simulink model "PreventOversaturationTest"  (R2025b)
settings: Solver=VariableStepAuto  StartTime=0.0  StopTime=10.0  RelTol=1e-3
libraries: Bibliothek_FHDO_V1 x7, simulink x1
settings Model: Creator=goessling  LastModifiedBy=goessling

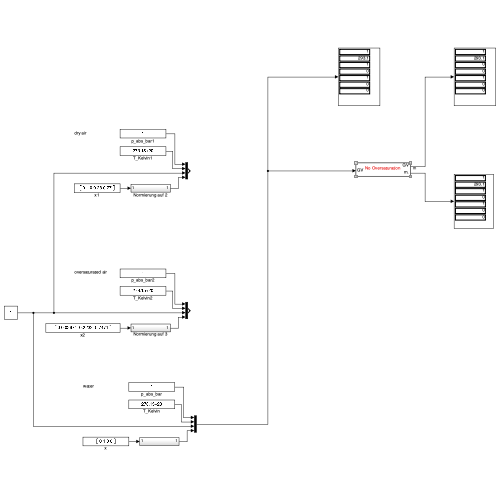
[thumbnail: Simulink's stored preview of the top-level diagram]
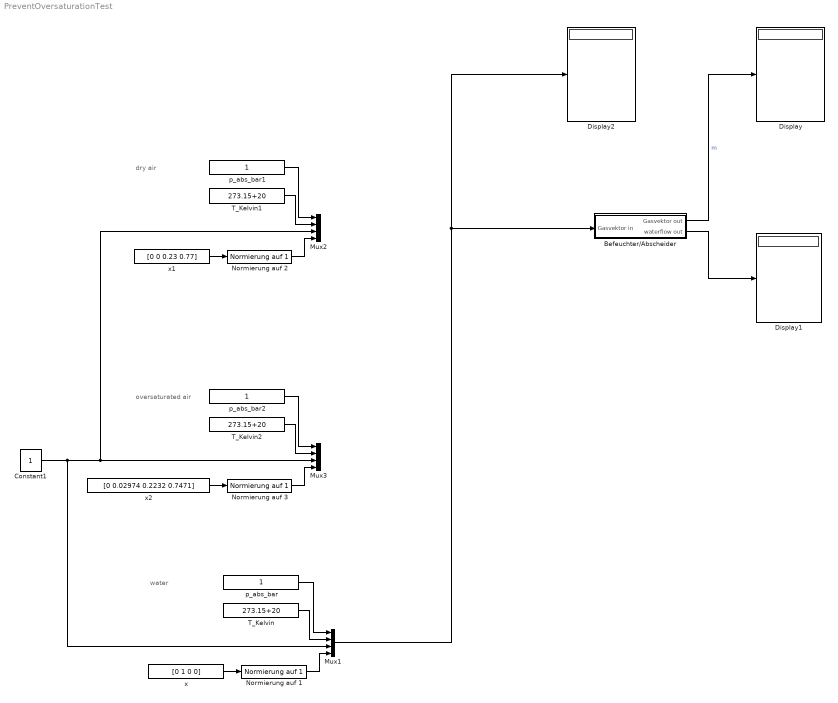
== system PreventOversaturationTest ==
  note: dry air
  note: oversaturated air
  note: water
  Befeuchter/Abscheider : Subsystem
      mask Display:
      | color('red')
      | disp('No Oversaturation');
      | 
      | color('black')
      | port_label('output', 1, 'GV')
      | port_label('output', 2, 'm.')
      | port_label('input', 1, 'GV')
  Constant1 : Constant
  Display : Display
  Display1 : Display
  Display2 : Display
  Mux1 : Mux
  Mux2 : Mux
  Mux3 : Mux
  Normierung auf 1 : Bibliothek_FHDO_V1/Wasser/Normierung auf 1  SystemSampleTime=-1  VariantActivationTime=update diagram  EmptyChoice=off  PassThrough=off  PassThroughVariantControl=(default)  EmptyChoiceVariantControl=(default)  AllowFlexibleInterface=on  Latency=0  AutoFrameSizeCalculation=off
  Normierung auf 2 : Bibliothek_FHDO_V1/Wasser/Normierung auf 1  SystemSampleTime=-1  VariantActivationTime=update diagram  EmptyChoice=off  PassThrough=off  PassThroughVariantControl=(default)  EmptyChoiceVariantControl=(default)  AllowFlexibleInterface=on  Latency=0  AutoFrameSizeCalculation=off
  Normierung auf 3 : Bibliothek_FHDO_V1/Wasser/Normierung auf 1  SystemSampleTime=-1  VariantActivationTime=update diagram  EmptyChoice=off  PassThrough=off  PassThroughVariantControl=(default)  EmptyChoiceVariantControl=(default)  AllowFlexibleInterface=on  Latency=0  AutoFrameSizeCalculation=off
  T_Kelvin : Constant  Value=273.15+20
  T_Kelvin1 : Constant  Value=273.15+20
  T_Kelvin2 : Constant  Value=273.15+20
  p_abs_bar : Constant
  p_abs_bar1 : Constant
  p_abs_bar2 : Constant
  x : Constant  Value=[0 1 0 0]
  x1 : Constant  Value=[0 0 0.23 0.77]
  x2 : Constant  Value=[0 0.02974 0.2232 0.7471]
  wires:
  Normierung auf 3/1 -> Mux3/4
  p_abs_bar2/1 -> Mux3/1
  T_Kelvin1/1 -> Mux2/2
  p_abs_bar1/1 -> Mux2/1
  Normierung auf 2/1 -> Mux2/4
  x1/1 -> Normierung auf 2/1
  T_Kelvin2/1 -> Mux3/2
  x2/1 -> Normierung auf 3/1
  Befeuchter/Abscheider/1(Gasvektor out) -> Display/1  "m"
  Befeuchter/Abscheider/2(waterflow out) -> Display1/1
  Normierung auf 1/1 -> Mux1/4
  T_Kelvin/1 -> Mux1/2
  p_abs_bar/1 -> Mux1/1
  Constant1/1 -> Mux1/3, Mux2/3, Mux3/3
  x/1 -> Normierung auf 1/1
  Mux1/1 -> Befeuchter/Abscheider/1(Gasvektor in), Display2/1

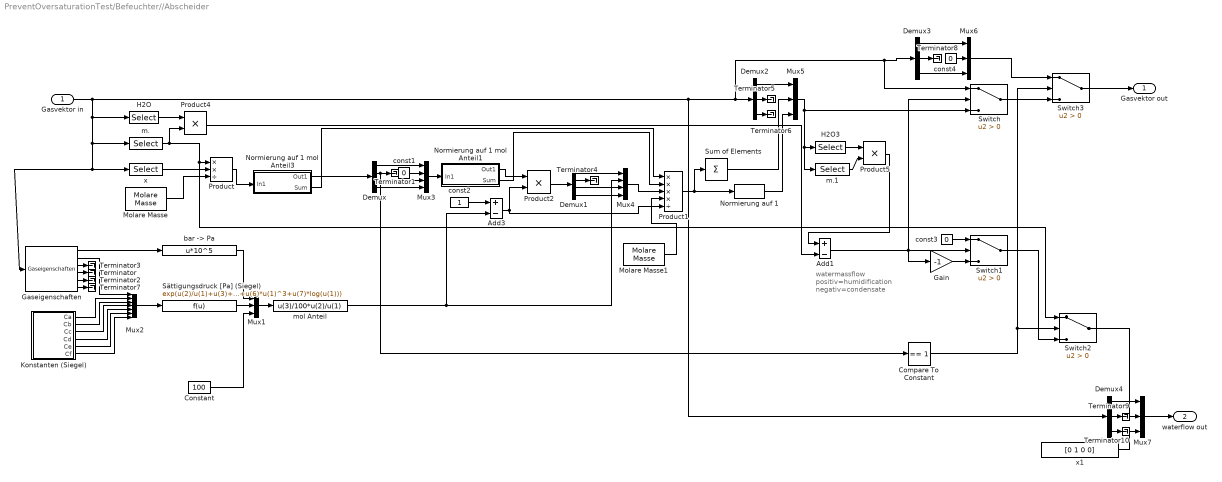
== system PreventOversaturationTest/Befeuchter//Abscheider ==
  note: watermassflow
      | positiv=humidification
      | negativ=condensate
  Gasvektor in : Inport
  Add1 : Sum  Inputs=+-
  Add3 : Sum  Inputs=+-
  Compare To Constant : simulink/Logic and Bit Operations/Compare To Constant  relop===  const=1  OutDataTypeStr=boolean
  Constant : Constant  Value=100
  Demux : Demux
  Demux1 : Demux
  Demux2 : Demux  Outputs=[2 1 4]
  Demux3 : Demux  Outputs=[2 1 4]
  Demux4 : Demux  Outputs=[2 1 4]
  Gain : Gain  Gain=-1
  Gaseigenschaften : Bibliothek_FHDO_V1/Gaseigenschaften  SystemSampleTime=-1  VariantActivationTime=update diagram  EmptyChoice=off  PassThrough=off  PassThroughVariantControl=(default)  EmptyChoiceVariantControl=(default)  AllowFlexibleInterface=on  Latency=0  AutoFrameSizeCalculation=off
  H2O : Selector  InputPortWidth=7  IndexOptions=Index vector (dialog)  Indices=5  OutputSizes=1
  H2O3 : Selector  InputPortWidth=7  IndexOptions=Index vector (dialog)  Indices=5  OutputSizes=1
  Konstanten (Siegel) : Subsystem
  Molare Masse : Bibliothek_FHDO_V1/Molare Masse  SystemSampleTime=-1  VariantActivationTime=update diagram  EmptyChoice=off  PassThrough=off  PassThroughVariantControl=(default)  EmptyChoiceVariantControl=(default)  AllowFlexibleInterface=on  Latency=0  AutoFrameSizeCalculation=off
  Molare Masse1 : Bibliothek_FHDO_V1/Molare Masse  SystemSampleTime=-1  VariantActivationTime=update diagram  EmptyChoice=off  PassThrough=off  PassThroughVariantControl=(default)  EmptyChoiceVariantControl=(default)  AllowFlexibleInterface=on  Latency=0  AutoFrameSizeCalculation=off
  Mux{1,5..7} (4 alike) : Mux  Inputs=3
  Mux2 : Mux  Inputs=7
  Mux3 : Mux
  Mux4 : Mux
  Normierung auf 1 : Bibliothek_FHDO_V1/Sauerstoff/Normierung auf 1  SystemSampleTime=-1  VariantActivationTime=update diagram  EmptyChoice=off  PassThrough=off  PassThroughVariantControl=(default)  EmptyChoiceVariantControl=(default)  AllowFlexibleInterface=on  Latency=0  AutoFrameSizeCalculation=off
  Normierung auf 1 mol Anteil1 : Subsystem
  Normierung auf 1 mol Anteil3 : Subsystem
  Product : Product  Inputs=**/  RndMeth=Zero
  Product1 : Product  Inputs=****/  RndMeth=Zero
  Product2 : Product  RndMeth=Zero
  Product4 : Product  RndMeth=Zero
  Product5 : Product  RndMeth=Zero
  Sum of Elements : Sum  Inputs=+
  Switch{,1..3} (4 alike) : Switch  Criteria=u2 > Threshold  SaturateOnIntegerOverflow=off  InputSameDT=off
  Sättigungsdruck [Pa] (Siegel) : Fcn  Expr=exp(u(2)/u(1)+u(3)+u(4)*u(1)+u(5)*u(1)^2+u(6)*u(1)^3+u(7)*log(u(1)))
  Terminator{,1..10} (11 alike) : Terminator
  "bar -> Pa" : Fcn  Expr=u*10^5
  const1 : Constant  Value=0
  const2 : Constant
  const3 : Constant  Value=0
  const4 : Constant  Value=0
  m. : Selector  InputPortWidth=7  IndexOptions=Index vector (dialog)  Indices=3  OutputSizes=1
  m.1 : Selector  InputPortWidth=7  IndexOptions=Index vector (dialog)  Indices=3  OutputSizes=1
  mol Anteil : Fcn  Expr=u(3)/100*u(2)/u(1)
  x : Selector  InputPortWidth=7  IndexOptions=Index vector (dialog)  Indices=[4 5 6 7]  OutputSizes=1
  x1 : Constant  Value=[0 1 0 0]
  Gasvektor out : Outport
  waterflow out : Outport  Port=2
  wires:
  Demux1/4 -> Mux4/4
  Demux1/3 -> Mux4/3
  Demux1/1 -> Mux4/1
  Demux1/2 -> Terminator4/1
  Demux/4 -> Mux3/4
  Demux/3 -> Mux3/3
  Demux/1 -> Mux3/1
  const1/1 -> Mux3/2
  Demux/2 -> Compare To Constant/1, Terminator1/1
  Product4/1 -> Add1/2
  Product5/1 -> Add1/1
  H2O3/1 -> Product5/1
  m.1/1 -> Product5/2
  H2O/1 -> Product4/1
  Normierung auf 1 mol Anteil1/2(Sum) -> Product1/2
  Normierung auf 1 mol Anteil3/2(Sum) -> Product1/1
  Normierung auf 1 mol Anteil3/1(Out1) -> Demux/1
  Normierung auf 1/1 -> Mux5/3
  Mux5/1 -> Switch/3, m.1/1, H2O3/1
  Demux2/3 -> Terminator6/1
  Demux2/2 -> Terminator5/1
  Product1/1 -> Normierung auf 1/1, Sum of Elements/1
  Sum of Elements/1 -> Mux5/2
  Demux2/1 -> Mux5/1
  m./1 -> Switch2/1, Product/1, Product4/2
  Molare Masse1/1 -> Product1/4
  Mux4/1 -> Product1/3
  Product2/1 -> Demux1/1
  Add3/1 -> Product1/5, Product2/2
  Normierung auf 1 mol Anteil1/1(Out1) -> Product2/1
  mol Anteil/1 -> Mux4/2, Add3/2
  const2/1 -> Add3/1
  Mux3/1 -> Normierung auf 1 mol Anteil1/1(In1)
  Product/1 -> Normierung auf 1 mol Anteil3/1(In1)
  Molare Masse/1 -> Product/3
  x/1 -> Product/2
  "bar -> Pa"/1 -> Mux1/1
  Constant/1 -> Mux1/3
  Mux1/1 -> mol Anteil/1
  Sättigungsdruck [Pa] (Siegel)/1 -> Mux1/2
  Mux2/1 -> Sättigungsdruck [Pa] (Siegel)/1
  Gaseigenschaften/5 -> Terminator2/1
  Gaseigenschaften/4 -> Terminator/1
  Gaseigenschaften/3 -> Terminator3/1
  Gaseigenschaften/1 -> "bar -> Pa"/1
  Konstanten (Siegel)/6(Cf) -> Mux2/7
  Konstanten (Siegel)/5(Ce) -> Mux2/6
  Konstanten (Siegel)/4(Cd) -> Mux2/5
  Konstanten (Siegel)/3(Cc) -> Mux2/4
  Konstanten (Siegel)/2(Cb) -> Mux2/3
  Konstanten (Siegel)/1(Ca) -> Mux2/2
  Gaseigenschaften/2 -> Mux2/1
  Gasvektor in/1 -> Demux3/1, Switch/1, Demux2/1, Demux4/1, H2O/1, Gaseigenschaften/1, x/1, m./1
  Gaseigenschaften/6 -> Terminator7/1
  Add1/1 -> Gain/1, Switch1/2, Switch/2
  Switch/1 -> Switch3/3
  const3/1 -> Switch1/1
  Compare To Constant/1 -> Switch3/2, Switch2/2
  Switch2/1 -> Mux7/2
  Switch1/1 -> Switch2/3
  Demux3/1 -> Mux6/1
  Demux3/3 -> Mux6/3
  const4/1 -> Mux6/2
  Demux3/2 -> Terminator8/1
  Mux6/1 -> Switch3/1
  Switch3/1 -> Gasvektor out/1
  Demux4/1 -> Mux7/1
  Demux4/2 -> Terminator9/1
  Demux4/3 -> Terminator10/1
  x1/1 -> Mux7/3
  Mux7/1 -> waterflow out/1
  Gain/1 -> Switch1/3

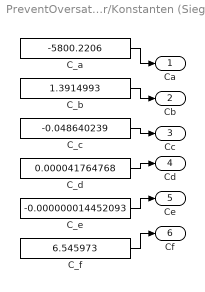
== system PreventOversaturationTest/Befeuchter//Abscheider/Konstanten (Siegel) ==
  C_a : Constant  Value=-5800.2206
  C_b : Constant  Value=1.3914993
  C_c : Constant  Value=-0.048640239
  C_d : Constant  Value=0.000041764768
  C_e : Constant  Value=-0.000000014452093
  C_f : Constant  Value=6.545973
  Ca : Outport
  Cb : Outport  Port=2
  Cc : Outport  Port=3
  Cd : Outport  Port=4
  Ce : Outport  Port=5
  Cf : Outport  Port=6
  wires:
  C_f/1 -> Cf/1
  C_e/1 -> Ce/1
  C_d/1 -> Cd/1
  C_c/1 -> Cc/1
  C_b/1 -> Cb/1
  C_a/1 -> Ca/1

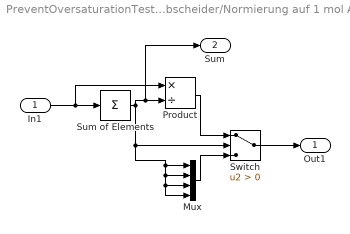
== system PreventOversaturationTest/Befeuchter//Abscheider/Normierung auf 1 mol Anteil1 ==
  In1 : Inport
  Mux : Mux
  Product : Product  Inputs=*/  RndMeth=Zero
  Sum of Elements : Sum  Inputs=+
  Switch : Switch  Criteria=u2 > Threshold  SaturateOnIntegerOverflow=off  InputSameDT=off
  Out1 : Outport
  Sum : Outport  Port=2
  wires:
  In1/1 -> Sum of Elements/1, Product/1
  Sum of Elements/1 -> Switch/2, Mux/4, Mux/3, Mux/2, Mux/1, Product/2, Sum/1
  Product/1 -> Switch/1
  Switch/1 -> Out1/1
  Mux/1 -> Switch/3

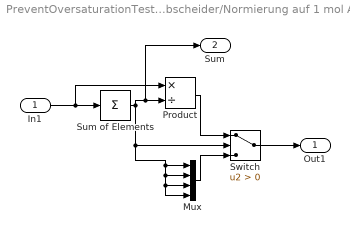
== system PreventOversaturationTest/Befeuchter//Abscheider/Normierung auf 1 mol Anteil3 ==
  In1 : Inport
  Mux : Mux
  Product : Product  Inputs=*/  RndMeth=Zero
  Sum of Elements : Sum  Inputs=+
  Switch : Switch  Criteria=u2 > Threshold  SaturateOnIntegerOverflow=off  InputSameDT=off
  Out1 : Outport
  Sum : Outport  Port=2
  wires:
  Mux/1 -> Switch/3
  Switch/1 -> Out1/1
  Product/1 -> Switch/1
  Sum of Elements/1 -> Sum/1, Product/2, Mux/1, Mux/2, Mux/3, Mux/4, Switch/2
  In1/1 -> Product/1, Sum of Elements/1
